simulink model "classB"  (Simulink 7.3)
settings: Solver=ode23tb  StartTime=0.0  StopTime=0.02  RelTol=1e-3
libraries: powerlib x9, powerlib_extras x2
settings Model: Creator=parthy  LastModifiedBy=srija
settings DebuggingCC: StrictBusMsg=ErrorLevel1

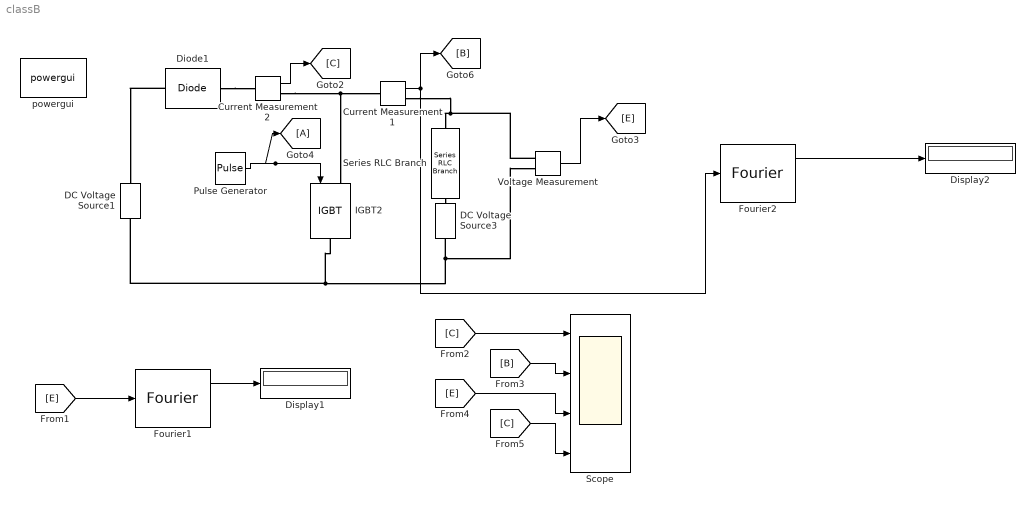
== system classB ==
  Current Measurement1 : powerlib/Measurements/Current Measurement  DialogController=POWERSYS.PowerSysDialog  SystemSampleTime=-1  PhasorSimulation=off  OutputType=Complex  PSBequivalent=0
  Current Measurement2 : powerlib/Measurements/Current Measurement  DialogController=POWERSYS.PowerSysDialog  SystemSampleTime=-1  PhasorSimulation=off  OutputType=Complex  PSBequivalent=0
  DC Voltage Source1 : powerlib/Electrical Sources/DC Voltage Source  DialogController=POWERSYS.PowerSysDialog  SystemSampleTime=-1  Amplitude=100  Measurements=None
  DC Voltage Source3 : powerlib/Electrical Sources/DC Voltage Source  DialogController=POWERSYS.PowerSysDialog  SystemSampleTime=-1  Amplitude=70  Measurements=None
  Diode1 : powerlib/Power Electronics/Diode  DialogController=POWERSYS.PowerSysDialog  SystemSampleTime=-1  Ron=0.001  Lon=0  Vf=0  IC=0  UseSnubber=off  Rs=500  Cs=250e-9  Measurements=off
  Display1 : Display
  Display2 : Display
  Fourier1 : powerlib_extras/Measurements/Fourier  DialogController=POWERSYS.PowerSysDialog  SystemSampleTime=-1  f1=1000  n=0
  Fourier2 : powerlib_extras/Measurements/Fourier  DialogController=POWERSYS.PowerSysDialog  SystemSampleTime=-1  f1=1000  n=0
  IGBT2 : powerlib/Power Electronics/IGBT  DialogController=POWERSYS.PowerSysDialog  SystemSampleTime=-1  Ron=0.001  Lon=0  Vf=0  Tf=1e-6  Tt=2e-6  IC=0  Rs=1e5  Cs=inf  Measurements=off
  Pulse Generator : DiscretePulseGenerator  PulseType=Time based  Amplitude=1  Period=1/1000  PulseWidth=0.0001  PhaseDelay=0  SampleTime=1
  Scope : Scope  NumInputPorts=4
      settings: YMin=0~-0.05~-10~-0.05  YMax=2~0.2~110~0.2
  Series RLC Branch : powerlib/Elements/Series RLC Branch  DialogController=POWERSYS.PowerSysDialog  PhysicalDomain=powersysdomain  SubClassName=unknown  LeftPortType=p1  RightPortType=p1  LConnTagsString=__new0  RConnTagsString=__new0  BranchType=RL  Resistance=10  Inductance=8e-3  SetiL0=off  InitialCurrent=0  Capacitance=1e-6  Setx0=off  InitialVoltage=0  Measurements=None
  Voltage Measurement : powerlib/Measurements/Voltage Measurement  DialogController=POWERSYS.PowerSysDialog  SystemSampleTime=-1  PhasorSimulation=off  OutputType=Complex  PSBequivalent=0
  powergui : powerlib/powergui  Priority=1  SystemSampleTime=-1  SimulationMode=Continuous  SampleTime=50e-6  frequency=60  SPID=on  DisableSnubberDevices=off  DisableRonSwitches=off  DisableVfSwitches=off  SwTol=0  Interpol=off  frequencyindice=0  echomessages=off  HookPort=off  DisplayEquations=off  FunctionMessages=off  EnableUseOfTLC=off  x0status=blocks  RestoreLinks=warning  Frange=[0:2:500]  Ylog=off  Xlog=on  ShowGrid=off  save=off  variable=ZData  ZoomFFT=on  StartTime=0.0  cycles=1  DisplayStyle=1  fundamental=60  FreqAxis=off  MaxFrequency=1000  frequencyindicesteady=1  RmsSteady=1  display=off  Ts=0  methode=off
  wires:
  Voltage Measurement/1 -> [E]
  [E] -> Fourier1/1
  Fourier1/1 -> Display1/1
  [C] -> Scope/1
  [B] -> Scope/2
  [E] -> Scope/3
  [C] -> Scope/4
  Pulse Generator/1 -> IGBT2/1, [A]
  Current Measurement1/1 -> [B], Fourier2/1
  Current Measurement2/1 -> [C]
  Fourier2/1 -> Display2/1
  connections:
  IGBT2/RConn1 -- Voltage Measurement/LConn2 -- DC Voltage Source3/LConn1 -- DC Voltage Source1/LConn1
  Current Measurement2/RConn1 -- IGBT2/LConn1 -- Current Measurement1/LConn1
  Series RLC Branch/RConn1 -- DC Voltage Source3/RConn1
  Voltage Measurement/LConn1 -- Series RLC Branch/LConn1 -- Current Measurement1/RConn1
  Diode1/LConn1 -- Current Measurement2/LConn1
  Diode1/RConn1 -- DC Voltage Source1/RConn1
